simulink model "Fig414"  (R2014b)
settings: Solver=FixedStepDiscrete  StartTime=0.0  StopTime=2  FixedStep=1e-3  RelTol=1e-3
libraries: simulink x3, commsrccod2 x2
settings Model: Creator=Dennis Silage  LastModifiedBy=Silage
settings DataIOCC: SignalLoggingSaveFormat=ModelDataLogs
settings OptimizationCC: ExpressionDepthLimit=2147483647  InitFltsAndDblsToZero=on
settings DebuggingCC: UnderspecifiedInitializationDetection=Classic  MergeDetectMultiDrivingBlocksExec=none  FcnCallInpInsideContextMsg=UseLocalSettings  StateNameClashWarn=warning
settings GRTTargetCC: CombineOutputUpdateFcns=off  GRTInterface=on

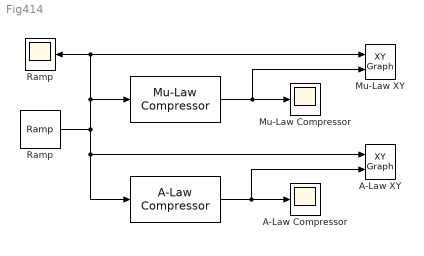
== system Fig414 ==
  " " : commsrccod2/Mu-Law Compressor  mu=255  V=1
  "   " : commsrccod2/A-Law Compressor  A=87.6  V=1
  A-Law Compressor : Scope
      settings: SaveName=ScopeData3
  A-Law XY : simulink/Sinks/XY Graph  xmin=-1  xmax=1  ymin=-1  ymax=1  st=-1
  Mu-Law Compressor : Scope
  Mu-Law XY : simulink/Sinks/XY Graph  xmin=-1  xmax=1  ymin=-1  ymax=1  st=-1
  Ramp : simulink/Sources/Ramp  slope=1  start=0  X0=-1
  "Ramp " : Scope
  wires:
  Ramp/1 -> "   "/1, A-Law XY/1, "Ramp "/1, Mu-Law XY/1, " "/1
  " "/1 -> Mu-Law XY/2, Mu-Law Compressor/1
  "   "/1 -> A-Law XY/2, A-Law Compressor/1
